simulink model "gg_plus_lc_platoon"  (R2019a)
settings: Solver=ode23t  StartTime=0.0  StopTime=70  FixedStep=0.1  MaxStep=0.01  RelTol=1e-3
InitFcn:
  | load vehStatesBus
libraries: simulink x120, powerlib_meascontrol x14, dspsigops x7, autolibshared x7
(part 6 of 7)

== system gg_plus_lc_platoon/Lo/Regular Vehicle Following/Compute Errors ==
  xf : Inport
  vf : Inport  Port=2
  xl : Inport  Port=3
  vl : Inport  Port=4
  extraSpaceFlag : Inport  Port=5
  velFilterReset : Inport  Port=6
  Compare To Constant : simulink/Logic and Bit Operations/Compare To Constant  relop=<  const=-0.1  OutDataTypeStr=boolean
  Demux : Demux  Outputs=2
  Demux1 : Demux  Outputs=2
  Gain3 : Gain  Gain=velFilterGain
  Integrator : Integrator  InitialCondition=[h d0]
  Integrator1 : Integrator  ExternalReset=rising  InitialCondition=vx0
  Multiply : Product
  Mux : Mux  Inputs=2
  Mux1 : Mux  Inputs=2
  Product : Product
  Saturation : Saturate  UpperLimit=maxAcceleration  LowerLimit=minAcceleration
  Saturation1 : Saturate  UpperLimit=hFilterSaturation  LowerLimit=-hFilterSaturation
  Sum : Sum  Inputs=-+|
  Sum1 : Sum  Inputs=++|
  Sum2 : Sum  Inputs=+-|
  Sum3 : Sum  Inputs=|++
  Sum4 : Sum  Inputs=-+|
  Sum5 : Sum  Inputs=|+-
  Sum6 : Sum  Inputs=+-|
  Sum7 : Sum  Inputs=|++
  Sum8 : Sum  Inputs=|+-
  Switch : Switch  Criteria=u2 > Threshold
  d0 : Constant  Value=d0
  d0Lc : Constant  Value=d0Lc
  h : Constant  Value=h
  hFilterGain : Gain  Gain=hFilterGain
  hLc : Constant  Value=hLc
  vLen : Constant  Value=lr+lf
  eh : Outport
  ev : Outport  Port=2
  "gap " : Outport  Port=3
  unsafeFlag : Outport  Port=4
  wires:
  Sum8/1 -> Gain3/1
  Integrator1/1 -> Sum4/2, Sum8/2
  Saturation/1 -> Integrator1/1
  Gain3/1 -> Saturation/1
  Sum4/1 -> ev/1
  vl/1 -> Sum8/1
  d0Lc/1 -> Mux1/2
  hFilterGain/1 -> Saturation1/1
  Demux/1 -> Multiply/2
  xf/1 -> Sum1/2
  Sum/1 -> Sum2/1, "gap "/1, Sum6/1  "gap"
  Multiply/1 -> Sum3/1
  Demux1/2 -> Sum7/2
  hLc/1 -> Mux1/1
  vLen/1 -> Sum1/1
  Demux/2 -> Sum3/2
  Switch/1 -> Sum5/1
  Sum5/1 -> hFilterGain/1
  vf/1 -> Multiply/1, Product/1, Sum4/1
  Sum1/1 -> Sum/1  "x (front bumber)"
  Sum3/1 -> Sum2/2  "desired  gap"
  h/1 -> Mux/1
  Product/1 -> Sum7/1
  xl/1 -> Sum/2
  extraSpaceFlag/1 -> Switch/2
  Sum2/1 -> eh/1
  Compare To Constant/1 -> unsafeFlag/1
  Demux1/1 -> Product/2
  Integrator/1 -> Sum5/2, Demux/1
  d0/1 -> Mux/2
  Mux1/1 -> Switch/1
  Sum7/1 -> Sum6/2  "safe  gap"
  Mux/1 -> Demux1/1, Switch/3  "min safe gap"
  Sum6/1 -> Compare To Constant/1
  velFilterReset/1 -> Integrator1/2
  Saturation1/1 -> Integrator/1

== system gg_plus_lc_platoon/Lo/Regular Vehicle Following/Veh Following ==
  eh : Inport
  ev : Inport  Port=2
  realInput : Inport  Port=3
  intReset : Inport  Port=4
  Anti-windup gain : Gain  Gain=sqrt(Ki/Kd)
  Integrator : Integrator  ExternalReset=rising
  Kd : Gain  Gain=Kd
  Ki : Gain  Gain=Ki
  Kp : Gain  Gain=Kp
  Saturation1 : Saturate  UpperLimit=maxHeadwayError  LowerLimit=minHeadwayError
  Scope : Scope  NumInputPorts=4
  Sum : Sum  Inputs=|-+
  Sum1 : Sum  Inputs=+++
  Sum5 : Sum  Inputs=-+|
  u : Outport
  wires:
  intReset/1 -> Integrator/2
  ev/1 -> Kd/1
  Ki/1 -> Sum5/2
  Anti-windup gain/1 -> Sum5/1
  Sum5/1 -> Integrator/1
  Kp/1 -> Sum1/2, Scope/2
  Kd/1 -> Sum1/3, Scope/3
  Saturation1/1 -> Ki/1, Kp/1
  eh/1 -> Saturation1/1
  Sum1/1 -> u/1, Sum/2, Scope/4
  realInput/1 -> Sum/1
  Sum/1 -> Anti-windup gain/1
  Integrator/1 -> Scope/1, Sum1/1

== system gg_plus_lc_platoon/Lo/Regular Vehicle Following/Velocity Control ==
  velocity : Inport
  realInput : Inport  Port=2
  intReset : Inport  Port=3
  Anti-windup gain : Gain  Gain=velKp/velKi
  Integrator2 : Integrator  ExternalReset=falling
  Sum : Sum  Inputs=|+-
  Sum1 : Sum  Inputs=|-+
  Sum2 : Sum  Inputs=-+|
  Sum3 : Sum  Inputs=|++
  freeFlowVel : Constant  Value=freeFlowVel
  velKi : Gain  Gain=velKi
  velKp : Gain  Gain=velKp
  u : Outport
  wires:
  Anti-windup gain/1 -> Sum2/1
  Sum/1 -> velKi/1, velKp/1
  velKp/1 -> Sum3/2
  velKi/1 -> Sum2/2
  Integrator2/1 -> Sum3/1
  velocity/1 -> Sum/2
  freeFlowVel/1 -> Sum/1
  intReset/1 -> Integrator2/2
  Sum3/1 -> Sum1/2, u/1
  realInput/1 -> Sum1/1
  Sum1/1 -> Anti-windup gain/1
  Sum2/1 -> Integrator2/1

== system gg_plus_lc_platoon/Lo/Subsystem1/Triggered Subsystem1 ==
  Trigger : TriggerPort  VariantControl=Variant
  Constant : Constant  Value=true  OutDataTypeStr=boolean
  Out1 : Outport  OutDataTypeStr=boolean  InitialOutput=0
  wires:
  Constant/1 -> Out1/1

== system gg_plus_lc_platoon/Lo/Subsystem1/safeErrors1 ==
  errors : Inport
  AND : Logic  IconShape=distinctive  AllPortsSameDT=off  OutDataTypeStr=boolean
  Compare To Constant4 : simulink/Logic and Bit Operations/Compare To Constant  relop=>=  const=-0.1  OutDataTypeStr=boolean
  Demux : Demux  Outputs=2
  safetyFlag : Outport
  wires:
  Compare To Constant4/1 -> Demux/1
  errors/1 -> Compare To Constant4/1
  AND/1 -> safetyFlag/1
  Demux/1 -> AND/1
  Demux/2 -> AND/2

== system gg_plus_lc_platoon/Lo/Subsystem1/safeErrors2 ==
  errors : Inport
  AND : Logic  IconShape=distinctive  AllPortsSameDT=off  OutDataTypeStr=boolean
  Compare To Constant4 : simulink/Logic and Bit Operations/Compare To Constant  relop=>=  const=-0.1  OutDataTypeStr=boolean
  Demux : Demux  Outputs=2
  safetyFlag : Outport
  wires:
  Demux/2 -> AND/2
  Demux/1 -> AND/1
  AND/1 -> safetyFlag/1
  errors/1 -> Compare To Constant4/1
  Compare To Constant4/1 -> Demux/1

== system gg_plus_lc_platoon/Lo/Subsystem1/steadyState ==
  u : Inport
  AND : Logic  IconShape=distinctive  AllPortsSameDT=off  OutDataTypeStr=boolean
  Abs2 : Abs
  Compare To Constant2 : simulink/Logic and Bit Operations/Compare To Constant  relop=<=  const=0.2  OutDataTypeStr=boolean
  Demux : Demux  Outputs=2
  Mux : Mux  Inputs=2
  Transport Delay2 : TransportDelay
  ssFlag : Outport
  wires:
  u/1 -> Transport Delay2/1, Mux/2
  Abs2/1 -> Compare To Constant2/1
  Demux/1 -> AND/1
  Transport Delay2/1 -> Mux/1
  AND/1 -> ssFlag/1
  Compare To Constant2/1 -> Demux/1
  Mux/1 -> Abs2/1
  Demux/2 -> AND/2

== system gg_plus_lc_platoon/Lo/Virtual Vehicle Following/Compute Errors ==
  xf : Inport
  vf : Inport  Port=2
  xl : Inport  Port=3
  vl : Inport  Port=4
  extraSpace : Inport  Port=5
  velFilterReset : Inport  Port=6
  Compare To Constant : simulink/Logic and Bit Operations/Compare To Constant  relop=<=  const=0  OutDataTypeStr=boolean
  Demux : Demux  Outputs=2
  Demux1 : Demux  Outputs=2
  Gain3 : Gain  Gain=velFilterGain/10
  Integrator : Integrator  InitialCondition=[h d0]
  Integrator1 : Integrator  ExternalReset=rising  InitialCondition=vx0
  Multiply : Product
  Mux : Mux  Inputs=2
  Mux1 : Mux  Inputs=2
  Product : Product
  Saturation : Saturate  UpperLimit=maxAcceleration  LowerLimit=minAcceleration
  Saturation1 : Saturate  UpperLimit=hFilterSaturation  LowerLimit=-hFilterSaturation
  Sum : Sum  Inputs=-+|
  Sum1 : Sum  Inputs=++|
  Sum2 : Sum  Inputs=+-|
  Sum3 : Sum  Inputs=|++
  Sum4 : Sum  Inputs=-+|
  Sum5 : Sum  Inputs=|+-
  Sum6 : Sum  Inputs=+-|
  Sum7 : Sum  Inputs=|++
  Sum8 : Sum  Inputs=|+-
  Switch : Switch  Criteria=u2 > Threshold
  d0 : Constant  Value=d0
  d0Lc : Constant  Value=d0Lc
  h : Constant  Value=h
  hFilterGain : Gain  Gain=hFilterGain
  hLc : Constant  Value=hLc
  vLen : Constant  Value=lr+lf
  eh : Outport
  ev : Outport  Port=2
  "gap " : Outport  Port=3
  unsafeFlag : Outport  Port=4
  wires:
  velFilterReset/1 -> Integrator1/2
  xl/1 -> Sum/2
  Sum6/1 -> Compare To Constant/1
  Mux/1 -> Demux1/1, Switch/3  "min safe gap"
  Sum7/1 -> Sum6/2  "safe  gap"
  Mux1/1 -> Switch/1
  d0/1 -> Mux/2
  Integrator/1 -> Demux/1, Sum5/2
  Demux1/1 -> Product/2
  Compare To Constant/1 -> unsafeFlag/1
  Sum2/1 -> eh/1
  extraSpace/1 -> Switch/2
  Product/1 -> Sum7/1
  h/1 -> Mux/1
  Sum3/1 -> Sum2/2  "desired  gap"
  Sum1/1 -> Sum/1  "x (front bumber)"
  vf/1 -> Sum4/1, Product/1, Multiply/1
  Sum5/1 -> hFilterGain/1
  Switch/1 -> Sum5/1
  Demux/2 -> Sum3/2
  vLen/1 -> Sum1/1
  hLc/1 -> Mux1/1
  Demux1/2 -> Sum7/2
  Multiply/1 -> Sum3/1
  Sum/1 -> Sum6/1, "gap "/1, Sum2/1  "gap"
  xf/1 -> Sum1/2
  Demux/1 -> Multiply/2
  hFilterGain/1 -> Saturation1/1
  d0Lc/1 -> Mux1/2
  Sum4/1 -> ev/1
  Integrator1/1 -> Sum4/2, Sum8/2
  Gain3/1 -> Saturation/1
  Sum8/1 -> Gain3/1
  Saturation/1 -> Integrator1/1
  vl/1 -> Sum8/1
  Saturation1/1 -> Integrator/1

== system gg_plus_lc_platoon/Lo/Virtual Vehicle Following/Velocity Control Free Flow ==
  ev : Inport
  realInput : Inport  Port=2
  intReset : Inport  Port=3
  Anti-windup gain : Gain  Gain=velKp/velKi
  Integrator2 : Integrator  ExternalReset=falling
  Sum1 : Sum  Inputs=|-+
  Sum2 : Sum  Inputs=-+|
  Sum3 : Sum  Inputs=|++
  velKi : Gain  Gain=velKi
  velKp : Gain  Gain=velKp
  u : Outport
  wires:
  Sum2/1 -> Integrator2/1
  Sum1/1 -> Anti-windup gain/1
  realInput/1 -> Sum1/1
  Anti-windup gain/1 -> Sum2/1
  Sum3/1 -> u/1, Sum1/2
  intReset/1 -> Integrator2/2
  Integrator2/1 -> Sum3/1
  velKi/1 -> Sum2/2
  velKp/1 -> Sum3/2
  ev/1 -> velKp/1, velKi/1

== system gg_plus_lc_platoon/Lo/Virtual Vehicle Following/Velocity Control Min ==
  note: Velocity control
  ev : Inport
  intReset : Inport  Port=2
  Integrator2 : Integrator  ExternalReset=rising
  Sum3 : Sum
  velKi : Gain  Gain=velKi
  velKp : Gain  Gain=velKp
  u : Outport
  wires:
  Integrator2/1 -> velKi/1
  velKi/1 -> Sum3/2
  Sum3/1 -> u/1
  velKp/1 -> Sum3/1
  ev/1 -> velKp/1, Integrator2/1
  intReset/1 -> Integrator2/2

== system gg_plus_lc_platoon/Lo/Virtual Vehicle Following/Virtual Leader Following ==
  eh : Inport
  ev : Inport  Port=2
  realInput : Inport  Port=3
  intReset : Inport  Port=4
  Anti-windup gain : Gain  Gain=sqrt(Ki/Kd)
  Gain : Gain  Gain=10
  Integrator : Integrator  ExternalReset=rising
  Integrator2 : Integrator  ExternalReset=rising
  Kd : Gain  Gain=Kd
  Ki : Gain  Gain=Ki
  Kp : Gain  Gain=Kp
  Saturation1 : Saturate  UpperLimit=maxHeadwayError  LowerLimit=minHeadwayError
  Scope : Scope  NumInputPorts=4
  Scope1 : Scope  NumInputPorts=2
  Sum : Sum  Inputs=|-+
  Sum1 : Sum  Inputs=+++
  Sum5 : Sum  Inputs=-+|
  Sum9 : Sum  Inputs=|+-
  u : Outport
  wires:
  Saturation1/1 -> Sum9/1, Scope1/1
  Sum9/1 -> Gain/1
  Gain/1 -> Integrator2/1
  ev/1 -> Kd/1
  Ki/1 -> Sum5/2
  Anti-windup gain/1 -> Sum5/1
  Sum5/1 -> Integrator/1
  Integrator/1 -> Sum1/1, Scope/1
  Kp/1 -> Scope/2, Sum1/2
  Kd/1 -> Scope/3, Sum1/3
  Integrator2/1 -> Kp/1, Ki/1, Scope1/2, Sum9/2
  eh/1 -> Saturation1/1
  Sum1/1 -> Sum/2, u/1, Scope/4
  realInput/1 -> Sum/1
  Sum/1 -> Anti-windup gain/1
  intReset/1 -> Integrator/2, Integrator2/2

== system gg_plus_lc_platoon/Lo/findLeader/Subsystem ==
  ego : Inport
  all : Inport  Port=2
  Enable : EnablePort
  MATLAB Function : MATLAB Function  TreatAsAtomicUnit=on
  idx : Outport  InitialOutput=1
  wires:
  ego/1 -> MATLAB Function/1(ego)
  MATLAB Function/1(leaderIdx) -> idx/1
  all/1 -> MATLAB Function/2(allVehicles)

== system gg_plus_lc_platoon/Lo/findLeader/farAwayVeh ==
  ego : Inport  OutDataTypeStr=Bus: vehStatesBus
  Bus Creator : BusCreator  Inputs=6  OutDataTypeStr=Bus: vehStatesBus  NonVirtualBus=on
  Bus Selector : BusSelector  OutputSignals=X,Y,Xdot,psi,u,delta
  Constant : Constant  Value=1000
  Sum : Sum  Inputs=++|
  Out1 : Outport  OutDataTypeStr=Bus: vehStatesBus
  wires:
  Bus Creator/1 -> Out1/1
  Constant/1 -> Sum/1
  Bus Selector/1 -> Sum/2  "<X>"
  ego/1 -> Bus Selector/1
  Sum/1 -> Bus Creator/1  "X"
  Bus Selector/2 -> Bus Creator/2  "<Y>"
  Bus Selector/3 -> Bus Creator/3  "<Xdot>"
  Bus Selector/4 -> Bus Creator/4  "<psi>"
  Bus Selector/5 -> Bus Creator/5  "<u>"
  Bus Selector/6 -> Bus Creator/6  "<delta>"

== system gg_plus_lc_platoon/Lo/followerErrors/gapToFollower ==
  xf : Inport
  vf : Inport  Port=2
  xl : Inport  Port=3
  Multiply : Product
  Sum : Sum  Inputs=-+|
  Sum1 : Sum  Inputs=++|
  Sum2 : Sum  Inputs=+-|
  Sum3 : Sum  Inputs=|++
  d0 : Constant  Value=d0
  h : Constant  Value=h
  vLen : Constant  Value=lr+lf
  eh : Outport
  "gap " : Outport  Port=2
  wires:
  vLen/1 -> Sum1/1
  Multiply/1 -> Sum3/1
  Sum/1 -> "gap "/1, Sum2/1  "gap"
  xf/1 -> Sum1/2
  Sum3/1 -> Sum2/2  "desired  gap"
  vf/1 -> Multiply/1
  Sum1/1 -> Sum/1  "x (front bumber)"
  xl/1 -> Sum/2
  Sum2/1 -> eh/1
  h/1 -> Multiply/2  "time headway"
  d0/1 -> Sum3/2  "gap at  standstill"

== system gg_plus_lc_platoon/Lo/safeErrors/Triggered Subsystem1 ==
  Trigger : TriggerPort  VariantControl=Variant
  Constant : Constant  Value=true  OutDataTypeStr=boolean
  Out1 : Outport  OutDataTypeStr=boolean  InitialOutput=0
  wires:
  Constant/1 -> Out1/1

== system gg_plus_lc_platoon/p1/Lateral Control/Full State Observer ==
  note: xhat
  note: yhat
  measuredOutputs : Inport
  delta : Inport  Port=2
  Add1 : Sum  Inputs=|-+
  Gain : Gain  Gain=B  Multiplication=Matrix(K*u)
  Gain1 : Gain  Gain=C  Multiplication=Matrix(K*u)
  Gain2 : Gain  Gain=L  Multiplication=Matrix(K*u)
  Gain3 : Gain  Gain=A  Multiplication=Matrix(K*u)
  Integrator : Integrator  InitialCondition=[y0; 0; 0; 0]
  Signal Specification : SignalSpecification  Dimensions=[size(C,1) 1]
  Sum : Sum  Inputs=+++
  xhat : Outport
  wires:
  Add1/1 -> Signal Specification/1
  Integrator/1 -> xhat/1, Gain3/1, Gain1/1
  Gain1/1 -> Add1/1
  Sum/1 -> Integrator/1
  measuredOutputs/1 -> Add1/2
  delta/1 -> Gain/1
  Gain/1 -> Sum/3
  Gain3/1 -> Sum/2
  Signal Specification/1 -> Gain2/1
  Gain2/1 -> Sum/1

== system gg_plus_lc_platoon/p1/Lateral Control/Triggered Subsystem1 ==
  In1 : Inport
  Trigger : TriggerPort  VariantControl=Variant
  Out1 : Outport  InitialOutput=y0
  wires:
  In1/1 -> Out1/1

== system gg_plus_lc_platoon/p1/Regular Vehicle Following/Compute Errors ==
  xf : Inport
  vf : Inport  Port=2
  xl : Inport  Port=3
  vl : Inport  Port=4
  extraSpaceFlag : Inport  Port=5
  velFilterReset : Inport  Port=6
  Compare To Constant : simulink/Logic and Bit Operations/Compare To Constant  relop=<  const=-0.1  OutDataTypeStr=boolean
  Demux : Demux  Outputs=2
  Demux1 : Demux  Outputs=2
  Gain3 : Gain  Gain=velFilterGain
  Integrator : Integrator  InitialCondition=[h d0]
  Integrator1 : Integrator  ExternalReset=rising  InitialCondition=vx0
  Multiply : Product
  Mux : Mux  Inputs=2
  Mux1 : Mux  Inputs=2
  Product : Product
  Saturation : Saturate  UpperLimit=maxAcceleration  LowerLimit=minAcceleration
  Saturation1 : Saturate  UpperLimit=hFilterSaturation  LowerLimit=-hFilterSaturation
  Sum : Sum  Inputs=-+|
  Sum1 : Sum  Inputs=++|
  Sum2 : Sum  Inputs=+-|
  Sum3 : Sum  Inputs=|++
  Sum4 : Sum  Inputs=-+|
  Sum5 : Sum  Inputs=|+-
  Sum6 : Sum  Inputs=+-|
  Sum7 : Sum  Inputs=|++
  Sum8 : Sum  Inputs=|+-
  Switch : Switch  Criteria=u2 > Threshold
  d0 : Constant  Value=d0
  d0Lc : Constant  Value=d0Lc
  h : Constant  Value=h
  hFilterGain : Gain  Gain=hFilterGain
  hLc : Constant  Value=hLc
  vLen : Constant  Value=lr+lf
  eh : Outport
  ev : Outport  Port=2
  "gap " : Outport  Port=3
  unsafeFlag : Outport  Port=4
  wires:
  Saturation1/1 -> Integrator/1
  velFilterReset/1 -> Integrator1/2
  Sum6/1 -> Compare To Constant/1
  Mux/1 -> Switch/3, Demux1/1  "min safe gap"
  Sum7/1 -> Sum6/2  "safe  gap"
  Mux1/1 -> Switch/1
  d0/1 -> Mux/2
  Integrator/1 -> Demux/1, Sum5/2
  Demux1/1 -> Product/2
  Compare To Constant/1 -> unsafeFlag/1
  Sum2/1 -> eh/1
  extraSpaceFlag/1 -> Switch/2
  xl/1 -> Sum/2
  Product/1 -> Sum7/1
  h/1 -> Mux/1
  Sum3/1 -> Sum2/2  "desired  gap"
  Sum1/1 -> Sum/1  "x (front bumber)"
  vf/1 -> Sum4/1, Product/1, Multiply/1
  Sum5/1 -> hFilterGain/1
  Switch/1 -> Sum5/1
  Demux/2 -> Sum3/2
  vLen/1 -> Sum1/1
  hLc/1 -> Mux1/1
  Demux1/2 -> Sum7/2
  Multiply/1 -> Sum3/1
  Sum/1 -> Sum6/1, "gap "/1, Sum2/1  "gap"
  xf/1 -> Sum1/2
  Demux/1 -> Multiply/2
  hFilterGain/1 -> Saturation1/1
  d0Lc/1 -> Mux1/2
  vl/1 -> Sum8/1
  Sum4/1 -> ev/1
  Gain3/1 -> Saturation/1
  Saturation/1 -> Integrator1/1
  Integrator1/1 -> Sum8/2, Sum4/2
  Sum8/1 -> Gain3/1

== system gg_plus_lc_platoon/p1/Regular Vehicle Following/Veh Following ==
  eh : Inport
  ev : Inport  Port=2
  realInput : Inport  Port=3
  intReset : Inport  Port=4
  Anti-windup gain : Gain  Gain=sqrt(Ki/Kd)
  Integrator : Integrator  ExternalReset=rising
  Kd : Gain  Gain=Kd
  Ki : Gain  Gain=Ki
  Kp : Gain  Gain=Kp
  Saturation1 : Saturate  UpperLimit=maxHeadwayError  LowerLimit=minHeadwayError
  Scope : Scope  NumInputPorts=4
  Sum : Sum  Inputs=|-+
  Sum1 : Sum  Inputs=+++
  Sum5 : Sum  Inputs=-+|
  u : Outport
  wires:
  Integrator/1 -> Sum1/1, Scope/1
  Sum/1 -> Anti-windup gain/1
  realInput/1 -> Sum/1
  Sum1/1 -> Scope/4, Sum/2, u/1
  eh/1 -> Saturation1/1
  Saturation1/1 -> Kp/1, Ki/1
  Kd/1 -> Scope/3, Sum1/3
  Kp/1 -> Scope/2, Sum1/2
  Sum5/1 -> Integrator/1
  Anti-windup gain/1 -> Sum5/1
  Ki/1 -> Sum5/2
  ev/1 -> Kd/1
  intReset/1 -> Integrator/2

== system gg_plus_lc_platoon/p1/Regular Vehicle Following/Velocity Control ==
  velocity : Inport
  realInput : Inport  Port=2
  intReset : Inport  Port=3
  Anti-windup gain : Gain  Gain=velKp/velKi
  Integrator2 : Integrator  ExternalReset=falling
  Sum : Sum  Inputs=|+-
  Sum1 : Sum  Inputs=|-+
  Sum2 : Sum  Inputs=-+|
  Sum3 : Sum  Inputs=|++
  freeFlowVel : Constant  Value=freeFlowVel
  velKi : Gain  Gain=velKi
  velKp : Gain  Gain=velKp
  u : Outport
  wires:
  Sum2/1 -> Integrator2/1
  Sum1/1 -> Anti-windup gain/1
  realInput/1 -> Sum1/1
  Sum3/1 -> u/1, Sum1/2
  intReset/1 -> Integrator2/2
  freeFlowVel/1 -> Sum/1
  velocity/1 -> Sum/2
  Integrator2/1 -> Sum3/1
  velKi/1 -> Sum2/2
  velKp/1 -> Sum3/2
  Sum/1 -> velKp/1, velKi/1
  Anti-windup gain/1 -> Sum2/1

== system gg_plus_lc_platoon/p1/Subsystem1/Triggered Subsystem1 ==
  Trigger : TriggerPort  VariantControl=Variant
  Constant : Constant  Value=true  OutDataTypeStr=boolean
  Out1 : Outport  OutDataTypeStr=boolean  InitialOutput=0
  wires:
  Constant/1 -> Out1/1

== system gg_plus_lc_platoon/p1/Subsystem1/safeErrors1 ==
  errors : Inport
  AND : Logic  IconShape=distinctive  AllPortsSameDT=off  OutDataTypeStr=boolean
  Compare To Constant4 : simulink/Logic and Bit Operations/Compare To Constant  relop=>=  const=-0.1  OutDataTypeStr=boolean
  Demux : Demux  Outputs=2
  safetyFlag : Outport
  wires:
  Demux/2 -> AND/2
  Demux/1 -> AND/1
  AND/1 -> safetyFlag/1
  errors/1 -> Compare To Constant4/1
  Compare To Constant4/1 -> Demux/1

== system gg_plus_lc_platoon/p1/Subsystem1/safeErrors2 ==
  errors : Inport
  AND : Logic  IconShape=distinctive  AllPortsSameDT=off  OutDataTypeStr=boolean
  Compare To Constant4 : simulink/Logic and Bit Operations/Compare To Constant  relop=>=  const=-0.1  OutDataTypeStr=boolean
  Demux : Demux  Outputs=2
  safetyFlag : Outport
  wires:
  Compare To Constant4/1 -> Demux/1
  errors/1 -> Compare To Constant4/1
  AND/1 -> safetyFlag/1
  Demux/1 -> AND/1
  Demux/2 -> AND/2

== system gg_plus_lc_platoon/p1/Subsystem1/steadyState ==
  u : Inport
  AND : Logic  IconShape=distinctive  AllPortsSameDT=off  OutDataTypeStr=boolean
  Abs2 : Abs
  Compare To Constant2 : simulink/Logic and Bit Operations/Compare To Constant  relop=<=  const=0.2  OutDataTypeStr=boolean
  Demux : Demux  Outputs=2
  Mux : Mux  Inputs=2
  Transport Delay2 : TransportDelay
  ssFlag : Outport
  wires:
  Demux/2 -> AND/2
  Mux/1 -> Abs2/1
  Compare To Constant2/1 -> Demux/1
  AND/1 -> ssFlag/1
  Transport Delay2/1 -> Mux/1
  Demux/1 -> AND/1
  Abs2/1 -> Compare To Constant2/1
  u/1 -> Mux/2, Transport Delay2/1

== system gg_plus_lc_platoon/p1/Virtual Vehicle Following/Compute Errors ==
  xf : Inport
  vf : Inport  Port=2
  xl : Inport  Port=3
  vl : Inport  Port=4
  extraSpace : Inport  Port=5
  velFilterReset : Inport  Port=6
  Compare To Constant : simulink/Logic and Bit Operations/Compare To Constant  relop=<=  const=0  OutDataTypeStr=boolean
  Demux : Demux  Outputs=2
  Demux1 : Demux  Outputs=2
  Gain3 : Gain  Gain=velFilterGain/10
  Integrator : Integrator  InitialCondition=[h d0]
  Integrator1 : Integrator  ExternalReset=rising  InitialCondition=vx0
  Multiply : Product
  Mux : Mux  Inputs=2
  Mux1 : Mux  Inputs=2
  Product : Product
  Saturation : Saturate  UpperLimit=maxAcceleration  LowerLimit=minAcceleration
  Saturation1 : Saturate  UpperLimit=hFilterSaturation  LowerLimit=-hFilterSaturation
  Sum : Sum  Inputs=-+|
  Sum1 : Sum  Inputs=++|
  Sum2 : Sum  Inputs=+-|
  Sum3 : Sum  Inputs=|++
  Sum4 : Sum  Inputs=-+|
  Sum5 : Sum  Inputs=|+-
  Sum6 : Sum  Inputs=+-|
  Sum7 : Sum  Inputs=|++
  Sum8 : Sum  Inputs=|+-
  Switch : Switch  Criteria=u2 > Threshold
  d0 : Constant  Value=d0
  d0Lc : Constant  Value=d0Lc
  h : Constant  Value=h
  hFilterGain : Gain  Gain=hFilterGain
  hLc : Constant  Value=hLc
  vLen : Constant  Value=lr+lf
  eh : Outport
  ev : Outport  Port=2
  "gap " : Outport  Port=3
  unsafeFlag : Outport  Port=4
  wires:
  Saturation1/1 -> Integrator/1
  vl/1 -> Sum8/1
  Saturation/1 -> Integrator1/1
  Sum8/1 -> Gain3/1
  Gain3/1 -> Saturation/1
  Integrator1/1 -> Sum8/2, Sum4/2
  Sum4/1 -> ev/1
  d0Lc/1 -> Mux1/2
  hFilterGain/1 -> Saturation1/1
  Demux/1 -> Multiply/2
  xf/1 -> Sum1/2
  Sum/1 -> Sum2/1, "gap "/1, Sum6/1  "gap"
  Multiply/1 -> Sum3/1
  Demux1/2 -> Sum7/2
  hLc/1 -> Mux1/1
  vLen/1 -> Sum1/1
  Demux/2 -> Sum3/2
  Switch/1 -> Sum5/1
  Sum5/1 -> hFilterGain/1
  vf/1 -> Multiply/1, Product/1, Sum4/1
  Sum1/1 -> Sum/1  "x (front bumber)"
  Sum3/1 -> Sum2/2  "desired  gap"
  h/1 -> Mux/1
  Product/1 -> Sum7/1
  extraSpace/1 -> Switch/2
  Sum2/1 -> eh/1
  Compare To Constant/1 -> unsafeFlag/1
  Demux1/1 -> Product/2
  Integrator/1 -> Sum5/2, Demux/1
  d0/1 -> Mux/2
  Mux1/1 -> Switch/1
  Sum7/1 -> Sum6/2  "safe  gap"
  Mux/1 -> Switch/3, Demux1/1  "min safe gap"
  Sum6/1 -> Compare To Constant/1
  xl/1 -> Sum/2
  velFilterReset/1 -> Integrator1/2

== system gg_plus_lc_platoon/p1/Virtual Vehicle Following/Velocity Control Free Flow ==
  ev : Inport
  realInput : Inport  Port=2
  intReset : Inport  Port=3
  Anti-windup gain : Gain  Gain=velKp/velKi
  Integrator2 : Integrator  ExternalReset=falling
  Sum1 : Sum  Inputs=|-+
  Sum2 : Sum  Inputs=-+|
  Sum3 : Sum  Inputs=|++
  velKi : Gain  Gain=velKi
  velKp : Gain  Gain=velKp
  u : Outport
  wires:
  ev/1 -> velKi/1, velKp/1
  velKp/1 -> Sum3/2
  velKi/1 -> Sum2/2
  Integrator2/1 -> Sum3/1
  intReset/1 -> Integrator2/2
  Sum3/1 -> Sum1/2, u/1
  Anti-windup gain/1 -> Sum2/1
  realInput/1 -> Sum1/1
  Sum1/1 -> Anti-windup gain/1
  Sum2/1 -> Integrator2/1

== system gg_plus_lc_platoon/p1/Virtual Vehicle Following/Velocity Control Min ==
  note: Velocity control
  ev : Inport
  intReset : Inport  Port=2
  Integrator2 : Integrator  ExternalReset=rising
  Sum3 : Sum
  velKi : Gain  Gain=velKi
  velKp : Gain  Gain=velKp
  u : Outport
  wires:
  intReset/1 -> Integrator2/2
  ev/1 -> Integrator2/1, velKp/1
  velKp/1 -> Sum3/1
  Sum3/1 -> u/1
  velKi/1 -> Sum3/2
  Integrator2/1 -> velKi/1

== system gg_plus_lc_platoon/p1/Virtual Vehicle Following/Virtual Leader Following ==
  eh : Inport
  ev : Inport  Port=2
  realInput : Inport  Port=3
  intReset : Inport  Port=4
  Anti-windup gain : Gain  Gain=sqrt(Ki/Kd)
  Gain : Gain  Gain=10
  Integrator : Integrator  ExternalReset=rising
  Integrator2 : Integrator  ExternalReset=rising
  Kd : Gain  Gain=Kd
  Ki : Gain  Gain=Ki
  Kp : Gain  Gain=Kp
  Saturation1 : Saturate  UpperLimit=maxHeadwayError  LowerLimit=minHeadwayError
  Scope : Scope  NumInputPorts=4
  Scope1 : Scope  NumInputPorts=2
  Sum : Sum  Inputs=|-+
  Sum1 : Sum  Inputs=+++
  Sum5 : Sum  Inputs=-+|
  Sum9 : Sum  Inputs=|+-
  u : Outport
  wires:
  intReset/1 -> Integrator2/2, Integrator/2
  Sum/1 -> Anti-windup gain/1
  realInput/1 -> Sum/1
  Sum1/1 -> Scope/4, u/1, Sum/2
  eh/1 -> Saturation1/1
  Integrator2/1 -> Sum9/2, Scope1/2, Ki/1, Kp/1
  Kd/1 -> Sum1/3, Scope/3
  Kp/1 -> Sum1/2, Scope/2
  Integrator/1 -> Scope/1, Sum1/1
  Sum5/1 -> Integrator/1
  Anti-windup gain/1 -> Sum5/1
  Ki/1 -> Sum5/2
  ev/1 -> Kd/1
  Gain/1 -> Integrator2/1
  Sum9/1 -> Gain/1
  Saturation1/1 -> Scope1/1, Sum9/1

== system gg_plus_lc_platoon/p1/findLeader/Subsystem ==
  ego : Inport
  all : Inport  Port=2
  Enable : EnablePort
  MATLAB Function : MATLAB Function  TreatAsAtomicUnit=on
  idx : Outport  InitialOutput=1
  wires:
  all/1 -> MATLAB Function/2(allVehicles)
  MATLAB Function/1(leaderIdx) -> idx/1
  ego/1 -> MATLAB Function/1(ego)

== system gg_plus_lc_platoon/p1/findLeader/farAwayVeh ==
  ego : Inport  OutDataTypeStr=Bus: vehStatesBus
  Bus Creator : BusCreator  Inputs=6  OutDataTypeStr=Bus: vehStatesBus  NonVirtualBus=on
  Bus Selector : BusSelector  OutputSignals=X,Y,Xdot,psi,u,delta
  Constant : Constant  Value=1000
  Sum : Sum  Inputs=++|
  Out1 : Outport  OutDataTypeStr=Bus: vehStatesBus
  wires:
  Bus Selector/6 -> Bus Creator/6  "<delta>"
  Bus Selector/5 -> Bus Creator/5  "<u>"
  Bus Selector/4 -> Bus Creator/4  "<psi>"
  Bus Selector/3 -> Bus Creator/3  "<Xdot>"
  Bus Selector/2 -> Bus Creator/2  "<Y>"
  Sum/1 -> Bus Creator/1  "X"
  ego/1 -> Bus Selector/1
  Bus Selector/1 -> Sum/2  "<X>"
  Constant/1 -> Sum/1
  Bus Creator/1 -> Out1/1

== system gg_plus_lc_platoon/p1/followerErrors/gapToFollower ==
  xf : Inport
  vf : Inport  Port=2
  xl : Inport  Port=3
  Multiply : Product
  Sum : Sum  Inputs=-+|
  Sum1 : Sum  Inputs=++|
  Sum2 : Sum  Inputs=+-|
  Sum3 : Sum  Inputs=|++
  d0 : Constant  Value=d0
  h : Constant  Value=h
  vLen : Constant  Value=lr+lf
  eh : Outport
  "gap " : Outport  Port=2
  wires:
  d0/1 -> Sum3/2  "gap at  standstill"
  h/1 -> Multiply/2  "time headway"
  Sum2/1 -> eh/1
  xl/1 -> Sum/2
  Sum1/1 -> Sum/1  "x (front bumber)"
  vf/1 -> Multiply/1
  Sum3/1 -> Sum2/2  "desired  gap"
  xf/1 -> Sum1/2
  Sum/1 -> Sum2/1, "gap "/1  "gap"
  Multiply/1 -> Sum3/1
  vLen/1 -> Sum1/1

== system gg_plus_lc_platoon/p1/safeErrors/Triggered Subsystem1 ==
  Trigger : TriggerPort  VariantControl=Variant
  Constant : Constant  Value=true  OutDataTypeStr=boolean
  Out1 : Outport  OutDataTypeStr=boolean  InitialOutput=0
  wires:
  Constant/1 -> Out1/1

== system gg_plus_lc_platoon/p2/Lateral Control/Full State Observer ==
  note: yhat
  note: xhat
  measuredOutputs : Inport
  delta : Inport  Port=2
  Add1 : Sum  Inputs=|-+
  Gain : Gain  Gain=B  Multiplication=Matrix(K*u)
  Gain1 : Gain  Gain=C  Multiplication=Matrix(K*u)
  Gain2 : Gain  Gain=L  Multiplication=Matrix(K*u)
  Gain3 : Gain  Gain=A  Multiplication=Matrix(K*u)
  Integrator : Integrator  InitialCondition=[y0; 0; 0; 0]
  Signal Specification : SignalSpecification  Dimensions=[size(C,1) 1]
  Sum : Sum  Inputs=+++
  xhat : Outport
  wires:
  Gain2/1 -> Sum/1
  Signal Specification/1 -> Gain2/1
  Gain3/1 -> Sum/2
  Gain/1 -> Sum/3
  delta/1 -> Gain/1
  measuredOutputs/1 -> Add1/2
  Sum/1 -> Integrator/1
  Gain1/1 -> Add1/1
  Integrator/1 -> Gain1/1, Gain3/1, xhat/1
  Add1/1 -> Signal Specification/1

== system gg_plus_lc_platoon/p2/Lateral Control/Triggered Subsystem1 ==
  In1 : Inport
  Trigger : TriggerPort  VariantControl=Variant
  Out1 : Outport  InitialOutput=y0
  wires:
  In1/1 -> Out1/1

== system gg_plus_lc_platoon/p2/Regular Vehicle Following/Compute Errors ==
  xf : Inport
  vf : Inport  Port=2
  xl : Inport  Port=3
  vl : Inport  Port=4
  extraSpaceFlag : Inport  Port=5
  velFilterReset : Inport  Port=6
  Compare To Constant : simulink/Logic and Bit Operations/Compare To Constant  relop=<  const=-0.1  OutDataTypeStr=boolean
  Demux : Demux  Outputs=2
  Demux1 : Demux  Outputs=2
  Gain3 : Gain  Gain=velFilterGain
  Integrator : Integrator  InitialCondition=[h d0]
  Integrator1 : Integrator  ExternalReset=rising  InitialCondition=vx0
  Multiply : Product
  Mux : Mux  Inputs=2
  Mux1 : Mux  Inputs=2
  Product : Product
  Saturation : Saturate  UpperLimit=maxAcceleration  LowerLimit=minAcceleration
  Saturation1 : Saturate  UpperLimit=hFilterSaturation  LowerLimit=-hFilterSaturation
  Sum : Sum  Inputs=-+|
  Sum1 : Sum  Inputs=++|
  Sum2 : Sum  Inputs=+-|
  Sum3 : Sum  Inputs=|++
  Sum4 : Sum  Inputs=-+|
  Sum5 : Sum  Inputs=|+-
  Sum6 : Sum  Inputs=+-|
  Sum7 : Sum  Inputs=|++
  Sum8 : Sum  Inputs=|+-
  Switch : Switch  Criteria=u2 > Threshold
  d0 : Constant  Value=d0
  d0Lc : Constant  Value=d0Lc
  h : Constant  Value=h
  hFilterGain : Gain  Gain=hFilterGain
  hLc : Constant  Value=hLc
  vLen : Constant  Value=lr+lf
  eh : Outport
  ev : Outport  Port=2
  "gap " : Outport  Port=3
  unsafeFlag : Outport  Port=4
  wires:
  Sum8/1 -> Gain3/1
  Integrator1/1 -> Sum4/2, Sum8/2
  Saturation/1 -> Integrator1/1
  Gain3/1 -> Saturation/1
  Sum4/1 -> ev/1
  vl/1 -> Sum8/1
  d0Lc/1 -> Mux1/2
  hFilterGain/1 -> Saturation1/1
  Demux/1 -> Multiply/2
  xf/1 -> Sum1/2
  Sum/1 -> Sum2/1, "gap "/1, Sum6/1  "gap"
  Multiply/1 -> Sum3/1
  Demux1/2 -> Sum7/2
  hLc/1 -> Mux1/1
  vLen/1 -> Sum1/1
  Demux/2 -> Sum3/2
  Switch/1 -> Sum5/1
  Sum5/1 -> hFilterGain/1
  vf/1 -> Multiply/1, Product/1, Sum4/1
  Sum1/1 -> Sum/1  "x (front bumber)"
  Sum3/1 -> Sum2/2  "desired  gap"
  h/1 -> Mux/1
  Product/1 -> Sum7/1
  xl/1 -> Sum/2
  extraSpaceFlag/1 -> Switch/2
  Sum2/1 -> eh/1
  Compare To Constant/1 -> unsafeFlag/1
  Demux1/1 -> Product/2
  Integrator/1 -> Sum5/2, Demux/1
  d0/1 -> Mux/2
  Mux1/1 -> Switch/1
  Sum7/1 -> Sum6/2  "safe  gap"
  Mux/1 -> Demux1/1, Switch/3  "min safe gap"
  Sum6/1 -> Compare To Constant/1
  velFilterReset/1 -> Integrator1/2
  Saturation1/1 -> Integrator/1

== system gg_plus_lc_platoon/p2/Regular Vehicle Following/Veh Following ==
  eh : Inport
  ev : Inport  Port=2
  realInput : Inport  Port=3
  intReset : Inport  Port=4
  Anti-windup gain : Gain  Gain=sqrt(Ki/Kd)
  Integrator : Integrator  ExternalReset=rising
  Kd : Gain  Gain=Kd
  Ki : Gain  Gain=Ki
  Kp : Gain  Gain=Kp
  Saturation1 : Saturate  UpperLimit=maxHeadwayError  LowerLimit=minHeadwayError
  Scope : Scope  NumInputPorts=4
  Sum : Sum  Inputs=|-+
  Sum1 : Sum  Inputs=+++
  Sum5 : Sum  Inputs=-+|
  u : Outport
  wires:
  intReset/1 -> Integrator/2
  ev/1 -> Kd/1
  Ki/1 -> Sum5/2
  Anti-windup gain/1 -> Sum5/1
  Sum5/1 -> Integrator/1
  Kp/1 -> Sum1/2, Scope/2
  Kd/1 -> Sum1/3, Scope/3
  Saturation1/1 -> Ki/1, Kp/1
  eh/1 -> Saturation1/1
  Sum1/1 -> u/1, Sum/2, Scope/4
  realInput/1 -> Sum/1
  Sum/1 -> Anti-windup gain/1
  Integrator/1 -> Scope/1, Sum1/1

== system gg_plus_lc_platoon/p2/Regular Vehicle Following/Velocity Control ==
  velocity : Inport
  realInput : Inport  Port=2
  intReset : Inport  Port=3
  Anti-windup gain : Gain  Gain=velKp/velKi
  Integrator2 : Integrator  ExternalReset=falling
  Sum : Sum  Inputs=|+-
  Sum1 : Sum  Inputs=|-+
  Sum2 : Sum  Inputs=-+|
  Sum3 : Sum  Inputs=|++
  freeFlowVel : Constant  Value=freeFlowVel
  velKi : Gain  Gain=velKi
  velKp : Gain  Gain=velKp
  u : Outport
  wires:
  Anti-windup gain/1 -> Sum2/1
  Sum/1 -> velKi/1, velKp/1
  velKp/1 -> Sum3/2
  velKi/1 -> Sum2/2
  Integrator2/1 -> Sum3/1
  velocity/1 -> Sum/2
  freeFlowVel/1 -> Sum/1
  intReset/1 -> Integrator2/2
  Sum3/1 -> Sum1/2, u/1
  realInput/1 -> Sum1/1
  Sum1/1 -> Anti-windup gain/1
  Sum2/1 -> Integrator2/1

== system gg_plus_lc_platoon/p2/Subsystem1/Triggered Subsystem1 ==
  Trigger : TriggerPort  VariantControl=Variant
  Constant : Constant  Value=true  OutDataTypeStr=boolean
  Out1 : Outport  OutDataTypeStr=boolean  InitialOutput=0
  wires:
  Constant/1 -> Out1/1

== system gg_plus_lc_platoon/p2/Subsystem1/safeErrors1 ==
  errors : Inport
  AND : Logic  IconShape=distinctive  AllPortsSameDT=off  OutDataTypeStr=boolean
  Compare To Constant4 : simulink/Logic and Bit Operations/Compare To Constant  relop=>=  const=-0.1  OutDataTypeStr=boolean
  Demux : Demux  Outputs=2
  safetyFlag : Outport
  wires:
  Compare To Constant4/1 -> Demux/1
  errors/1 -> Compare To Constant4/1
  AND/1 -> safetyFlag/1
  Demux/1 -> AND/1
  Demux/2 -> AND/2

== system gg_plus_lc_platoon/p2/Subsystem1/safeErrors2 ==
  errors : Inport
  AND : Logic  IconShape=distinctive  AllPortsSameDT=off  OutDataTypeStr=boolean
  Compare To Constant4 : simulink/Logic and Bit Operations/Compare To Constant  relop=>=  const=-0.1  OutDataTypeStr=boolean
  Demux : Demux  Outputs=2
  safetyFlag : Outport
  wires:
  Demux/2 -> AND/2
  Demux/1 -> AND/1
  AND/1 -> safetyFlag/1
  errors/1 -> Compare To Constant4/1
  Compare To Constant4/1 -> Demux/1

== system gg_plus_lc_platoon/p2/Subsystem1/steadyState ==
  u : Inport
  AND : Logic  IconShape=distinctive  AllPortsSameDT=off  OutDataTypeStr=boolean
  Abs2 : Abs
  Compare To Constant2 : simulink/Logic and Bit Operations/Compare To Constant  relop=<=  const=0.2  OutDataTypeStr=boolean
  Demux : Demux  Outputs=2
  Mux : Mux  Inputs=2
  Transport Delay2 : TransportDelay
  ssFlag : Outport
  wires:
  u/1 -> Transport Delay2/1, Mux/2
  Abs2/1 -> Compare To Constant2/1
  Demux/1 -> AND/1
  Transport Delay2/1 -> Mux/1
  AND/1 -> ssFlag/1
  Compare To Constant2/1 -> Demux/1
  Mux/1 -> Abs2/1
  Demux/2 -> AND/2

== system gg_plus_lc_platoon/p2/Virtual Vehicle Following/Compute Errors ==
  xf : Inport
  vf : Inport  Port=2
  xl : Inport  Port=3
  vl : Inport  Port=4
  extraSpace : Inport  Port=5
  velFilterReset : Inport  Port=6
  Compare To Constant : simulink/Logic and Bit Operations/Compare To Constant  relop=<=  const=0  OutDataTypeStr=boolean
  Demux : Demux  Outputs=2
  Demux1 : Demux  Outputs=2
  Gain3 : Gain  Gain=velFilterGain/10
  Integrator : Integrator  InitialCondition=[h d0]
  Integrator1 : Integrator  ExternalReset=rising  InitialCondition=vx0
  Multiply : Product
  Mux : Mux  Inputs=2
  Mux1 : Mux  Inputs=2
  Product : Product
  Saturation : Saturate  UpperLimit=maxAcceleration  LowerLimit=minAcceleration
  Saturation1 : Saturate  UpperLimit=hFilterSaturation  LowerLimit=-hFilterSaturation
  Sum : Sum  Inputs=-+|
  Sum1 : Sum  Inputs=++|
  Sum2 : Sum  Inputs=+-|
  Sum3 : Sum  Inputs=|++
  Sum4 : Sum  Inputs=-+|
  Sum5 : Sum  Inputs=|+-
  Sum6 : Sum  Inputs=+-|
  Sum7 : Sum  Inputs=|++
  Sum8 : Sum  Inputs=|+-
  Switch : Switch  Criteria=u2 > Threshold
  d0 : Constant  Value=d0
  d0Lc : Constant  Value=d0Lc
  h : Constant  Value=h
  hFilterGain : Gain  Gain=hFilterGain
  hLc : Constant  Value=hLc
  vLen : Constant  Value=lr+lf
  eh : Outport
  ev : Outport  Port=2
  "gap " : Outport  Port=3
  unsafeFlag : Outport  Port=4
  wires:
  velFilterReset/1 -> Integrator1/2
  xl/1 -> Sum/2
  Sum6/1 -> Compare To Constant/1
  Mux/1 -> Demux1/1, Switch/3  "min safe gap"
  Sum7/1 -> Sum6/2  "safe  gap"
  Mux1/1 -> Switch/1
  d0/1 -> Mux/2
  Integrator/1 -> Demux/1, Sum5/2
  Demux1/1 -> Product/2
  Compare To Constant/1 -> unsafeFlag/1
  Sum2/1 -> eh/1
  extraSpace/1 -> Switch/2
  Product/1 -> Sum7/1
  h/1 -> Mux/1
  Sum3/1 -> Sum2/2  "desired  gap"
  Sum1/1 -> Sum/1  "x (front bumber)"
  vf/1 -> Sum4/1, Product/1, Multiply/1
  Sum5/1 -> hFilterGain/1
  Switch/1 -> Sum5/1
  Demux/2 -> Sum3/2
  vLen/1 -> Sum1/1
  hLc/1 -> Mux1/1
  Demux1/2 -> Sum7/2
  Multiply/1 -> Sum3/1
  Sum/1 -> Sum6/1, "gap "/1, Sum2/1  "gap"
  xf/1 -> Sum1/2
  Demux/1 -> Multiply/2
  hFilterGain/1 -> Saturation1/1
  d0Lc/1 -> Mux1/2
  Sum4/1 -> ev/1
  Integrator1/1 -> Sum4/2, Sum8/2
  Gain3/1 -> Saturation/1
  Sum8/1 -> Gain3/1
  Saturation/1 -> Integrator1/1
  vl/1 -> Sum8/1
  Saturation1/1 -> Integrator/1

== system gg_plus_lc_platoon/p2/Virtual Vehicle Following/Velocity Control Free Flow ==
  ev : Inport
  realInput : Inport  Port=2
  intReset : Inport  Port=3
  Anti-windup gain : Gain  Gain=velKp/velKi
  Integrator2 : Integrator  ExternalReset=falling
  Sum1 : Sum  Inputs=|-+
  Sum2 : Sum  Inputs=-+|
  Sum3 : Sum  Inputs=|++
  velKi : Gain  Gain=velKi
  velKp : Gain  Gain=velKp
  u : Outport
  wires:
  Sum2/1 -> Integrator2/1
  Sum1/1 -> Anti-windup gain/1
  realInput/1 -> Sum1/1
  Anti-windup gain/1 -> Sum2/1
  Sum3/1 -> u/1, Sum1/2
  intReset/1 -> Integrator2/2
  Integrator2/1 -> Sum3/1
  velKi/1 -> Sum2/2
  velKp/1 -> Sum3/2
  ev/1 -> velKp/1, velKi/1

== system gg_plus_lc_platoon/p2/Virtual Vehicle Following/Velocity Control Min ==
  note: Velocity control
  ev : Inport
  intReset : Inport  Port=2
  Integrator2 : Integrator  ExternalReset=rising
  Sum3 : Sum
  velKi : Gain  Gain=velKi
  velKp : Gain  Gain=velKp
  u : Outport
  wires:
  Integrator2/1 -> velKi/1
  velKi/1 -> Sum3/2
  Sum3/1 -> u/1
  velKp/1 -> Sum3/1
  ev/1 -> velKp/1, Integrator2/1
  intReset/1 -> Integrator2/2

== system gg_plus_lc_platoon/p2/Virtual Vehicle Following/Virtual Leader Following ==
  eh : Inport
  ev : Inport  Port=2
  realInput : Inport  Port=3
  intReset : Inport  Port=4
  Anti-windup gain : Gain  Gain=sqrt(Ki/Kd)
  Gain : Gain  Gain=10
  Integrator : Integrator  ExternalReset=rising
  Integrator2 : Integrator  ExternalReset=rising
  Kd : Gain  Gain=Kd
  Ki : Gain  Gain=Ki
  Kp : Gain  Gain=Kp
  Saturation1 : Saturate  UpperLimit=maxHeadwayError  LowerLimit=minHeadwayError
  Scope : Scope  NumInputPorts=4
  Scope1 : Scope  NumInputPorts=2
  Sum : Sum  Inputs=|-+
  Sum1 : Sum  Inputs=+++
  Sum5 : Sum  Inputs=-+|
  Sum9 : Sum  Inputs=|+-
  u : Outport
  wires:
  Saturation1/1 -> Sum9/1, Scope1/1
  Sum9/1 -> Gain/1
  Gain/1 -> Integrator2/1
  ev/1 -> Kd/1
  Ki/1 -> Sum5/2
  Anti-windup gain/1 -> Sum5/1
  Sum5/1 -> Integrator/1
  Integrator/1 -> Sum1/1, Scope/1
  Kp/1 -> Scope/2, Sum1/2
  Kd/1 -> Scope/3, Sum1/3
  Integrator2/1 -> Kp/1, Ki/1, Scope1/2, Sum9/2
  eh/1 -> Saturation1/1
  Sum1/1 -> Sum/2, u/1, Scope/4
  realInput/1 -> Sum/1
  Sum/1 -> Anti-windup gain/1
  intReset/1 -> Integrator/2, Integrator2/2

== system gg_plus_lc_platoon/p2/findLeader/Subsystem ==
  ego : Inport
  all : Inport  Port=2
  Enable : EnablePort
  MATLAB Function : MATLAB Function  TreatAsAtomicUnit=on
  idx : Outport  InitialOutput=1
  wires:
  ego/1 -> MATLAB Function/1(ego)
  MATLAB Function/1(leaderIdx) -> idx/1
  all/1 -> MATLAB Function/2(allVehicles)

== system gg_plus_lc_platoon/p2/findLeader/farAwayVeh ==
  ego : Inport  OutDataTypeStr=Bus: vehStatesBus
  Bus Creator : BusCreator  Inputs=6  OutDataTypeStr=Bus: vehStatesBus  NonVirtualBus=on
  Bus Selector : BusSelector  OutputSignals=X,Y,Xdot,psi,u,delta
  Constant : Constant  Value=1000
  Sum : Sum  Inputs=++|
  Out1 : Outport  OutDataTypeStr=Bus: vehStatesBus
  wires:
  Bus Creator/1 -> Out1/1
  Constant/1 -> Sum/1
  Bus Selector/1 -> Sum/2  "<X>"
  ego/1 -> Bus Selector/1
  Sum/1 -> Bus Creator/1  "X"
  Bus Selector/2 -> Bus Creator/2  "<Y>"
  Bus Selector/3 -> Bus Creator/3  "<Xdot>"
  Bus Selector/4 -> Bus Creator/4  "<psi>"
  Bus Selector/5 -> Bus Creator/5  "<u>"
  Bus Selector/6 -> Bus Creator/6  "<delta>"

== system gg_plus_lc_platoon/p2/followerErrors/gapToFollower ==
  xf : Inport
  vf : Inport  Port=2
  xl : Inport  Port=3
  Multiply : Product
  Sum : Sum  Inputs=-+|
  Sum1 : Sum  Inputs=++|
  Sum2 : Sum  Inputs=+-|
  Sum3 : Sum  Inputs=|++
  d0 : Constant  Value=d0
  h : Constant  Value=h
  vLen : Constant  Value=lr+lf
  eh : Outport
  "gap " : Outport  Port=2
  wires:
  vLen/1 -> Sum1/1
  Multiply/1 -> Sum3/1
  Sum/1 -> "gap "/1, Sum2/1  "gap"
  xf/1 -> Sum1/2
  Sum3/1 -> Sum2/2  "desired  gap"
  vf/1 -> Multiply/1
  Sum1/1 -> Sum/1  "x (front bumber)"
  xl/1 -> Sum/2
  Sum2/1 -> eh/1
  h/1 -> Multiply/2  "time headway"
  d0/1 -> Sum3/2  "gap at  standstill"

== system gg_plus_lc_platoon/p2/safeErrors/Triggered Subsystem1 ==
  Trigger : TriggerPort  VariantControl=Variant
  Constant : Constant  Value=true  OutDataTypeStr=boolean
  Out1 : Outport  OutDataTypeStr=boolean  InitialOutput=0
  wires:
  Constant/1 -> Out1/1

== system gg_plus_lc_platoon/p3/Lateral Control/Full State Observer ==
  note: yhat
  note: xhat
  measuredOutputs : Inport
  delta : Inport  Port=2
  Add1 : Sum  Inputs=|-+
  Gain : Gain  Gain=B  Multiplication=Matrix(K*u)
  Gain1 : Gain  Gain=C  Multiplication=Matrix(K*u)
  Gain2 : Gain  Gain=L  Multiplication=Matrix(K*u)
  Gain3 : Gain  Gain=A  Multiplication=Matrix(K*u)
  Integrator : Integrator  InitialCondition=[y0; 0; 0; 0]
  Signal Specification : SignalSpecification  Dimensions=[size(C,1) 1]
  Sum : Sum  Inputs=+++
  xhat : Outport
  wires:
  Gain2/1 -> Sum/1
  Signal Specification/1 -> Gain2/1
  Gain3/1 -> Sum/2
  Gain/1 -> Sum/3
  delta/1 -> Gain/1
  measuredOutputs/1 -> Add1/2
  Sum/1 -> Integrator/1
  Gain1/1 -> Add1/1
  Integrator/1 -> Gain1/1, Gain3/1, xhat/1
  Add1/1 -> Signal Specification/1

== system gg_plus_lc_platoon/p3/Lateral Control/Triggered Subsystem1 ==
  In1 : Inport
  Trigger : TriggerPort  VariantControl=Variant
  Out1 : Outport  InitialOutput=y0
  wires:
  In1/1 -> Out1/1

== system gg_plus_lc_platoon/p3/Regular Vehicle Following/Compute Errors ==
  xf : Inport
  vf : Inport  Port=2
  xl : Inport  Port=3
  vl : Inport  Port=4
  extraSpaceFlag : Inport  Port=5
  velFilterReset : Inport  Port=6
  Compare To Constant : simulink/Logic and Bit Operations/Compare To Constant  relop=<  const=-0.1  OutDataTypeStr=boolean
  Demux : Demux  Outputs=2
  Demux1 : Demux  Outputs=2
  Gain3 : Gain  Gain=velFilterGain
  Integrator : Integrator  InitialCondition=[h d0]
  Integrator1 : Integrator  ExternalReset=rising  InitialCondition=vx0
  Multiply : Product
  Mux : Mux  Inputs=2
  Mux1 : Mux  Inputs=2
  Product : Product
  Saturation : Saturate  UpperLimit=maxAcceleration  LowerLimit=minAcceleration
  Saturation1 : Saturate  UpperLimit=hFilterSaturation  LowerLimit=-hFilterSaturation
  Sum : Sum  Inputs=-+|
  Sum1 : Sum  Inputs=++|
  Sum2 : Sum  Inputs=+-|
  Sum3 : Sum  Inputs=|++
  Sum4 : Sum  Inputs=-+|
  Sum5 : Sum  Inputs=|+-
  Sum6 : Sum  Inputs=+-|
  Sum7 : Sum  Inputs=|++
  Sum8 : Sum  Inputs=|+-
  Switch : Switch  Criteria=u2 > Threshold
  d0 : Constant  Value=d0
  d0Lc : Constant  Value=d0Lc
  h : Constant  Value=h
  hFilterGain : Gain  Gain=hFilterGain
  hLc : Constant  Value=hLc
  vLen : Constant  Value=lr+lf
  eh : Outport
  ev : Outport  Port=2
  "gap " : Outport  Port=3
  unsafeFlag : Outport  Port=4
  wires:
  Sum8/1 -> Gain3/1
  Integrator1/1 -> Sum4/2, Sum8/2
  Saturation/1 -> Integrator1/1
  Gain3/1 -> Saturation/1
  Sum4/1 -> ev/1
  vl/1 -> Sum8/1
  d0Lc/1 -> Mux1/2
  hFilterGain/1 -> Saturation1/1
  Demux/1 -> Multiply/2
  xf/1 -> Sum1/2
  Sum/1 -> Sum2/1, "gap "/1, Sum6/1  "gap"
  Multiply/1 -> Sum3/1
  Demux1/2 -> Sum7/2
  hLc/1 -> Mux1/1
  vLen/1 -> Sum1/1
  Demux/2 -> Sum3/2
  Switch/1 -> Sum5/1
  Sum5/1 -> hFilterGain/1
  vf/1 -> Multiply/1, Product/1, Sum4/1
  Sum1/1 -> Sum/1  "x (front bumber)"
  Sum3/1 -> Sum2/2  "desired  gap"
  h/1 -> Mux/1
  Product/1 -> Sum7/1
  xl/1 -> Sum/2
  extraSpaceFlag/1 -> Switch/2
  Sum2/1 -> eh/1
  Compare To Constant/1 -> unsafeFlag/1
  Demux1/1 -> Product/2
  Integrator/1 -> Sum5/2, Demux/1
  d0/1 -> Mux/2
  Mux1/1 -> Switch/1
  Sum7/1 -> Sum6/2  "safe  gap"
  Mux/1 -> Demux1/1, Switch/3  "min safe gap"
  Sum6/1 -> Compare To Constant/1
  velFilterReset/1 -> Integrator1/2
  Saturation1/1 -> Integrator/1

== system gg_plus_lc_platoon/p3/Regular Vehicle Following/Veh Following ==
  eh : Inport
  ev : Inport  Port=2
  realInput : Inport  Port=3
  intReset : Inport  Port=4
  Anti-windup gain : Gain  Gain=sqrt(Ki/Kd)
  Integrator : Integrator  ExternalReset=rising
  Kd : Gain  Gain=Kd
  Ki : Gain  Gain=Ki
  Kp : Gain  Gain=Kp
  Saturation1 : Saturate  UpperLimit=maxHeadwayError  LowerLimit=minHeadwayError
  Scope : Scope  NumInputPorts=4
  Sum : Sum  Inputs=|-+
  Sum1 : Sum  Inputs=+++
  Sum5 : Sum  Inputs=-+|
  u : Outport
  wires:
  intReset/1 -> Integrator/2
  ev/1 -> Kd/1
  Ki/1 -> Sum5/2
  Anti-windup gain/1 -> Sum5/1
  Sum5/1 -> Integrator/1
  Kp/1 -> Sum1/2, Scope/2
  Kd/1 -> Sum1/3, Scope/3
  Saturation1/1 -> Ki/1, Kp/1
  eh/1 -> Saturation1/1
  Sum1/1 -> u/1, Sum/2, Scope/4
  realInput/1 -> Sum/1
  Sum/1 -> Anti-windup gain/1
  Integrator/1 -> Scope/1, Sum1/1

== system gg_plus_lc_platoon/p3/Regular Vehicle Following/Velocity Control ==
  velocity : Inport
  realInput : Inport  Port=2
  intReset : Inport  Port=3
  Anti-windup gain : Gain  Gain=velKp/velKi
  Integrator2 : Integrator  ExternalReset=falling
  Sum : Sum  Inputs=|+-
  Sum1 : Sum  Inputs=|-+
  Sum2 : Sum  Inputs=-+|
  Sum3 : Sum  Inputs=|++
  freeFlowVel : Constant  Value=freeFlowVel
  velKi : Gain  Gain=velKi
  velKp : Gain  Gain=velKp
  u : Outport
  wires:
  Anti-windup gain/1 -> Sum2/1
  Sum/1 -> velKi/1, velKp/1
  velKp/1 -> Sum3/2
  velKi/1 -> Sum2/2
  Integrator2/1 -> Sum3/1
  velocity/1 -> Sum/2
  freeFlowVel/1 -> Sum/1
  intReset/1 -> Integrator2/2
  Sum3/1 -> Sum1/2, u/1
  realInput/1 -> Sum1/1
  Sum1/1 -> Anti-windup gain/1
  Sum2/1 -> Integrator2/1

== system gg_plus_lc_platoon/p3/Subsystem1/Triggered Subsystem1 ==
  Trigger : TriggerPort  VariantControl=Variant
  Constant : Constant  Value=true  OutDataTypeStr=boolean
  Out1 : Outport  OutDataTypeStr=boolean  InitialOutput=0
  wires:
  Constant/1 -> Out1/1

== system gg_plus_lc_platoon/p3/Subsystem1/safeErrors1 ==
  errors : Inport
  AND : Logic  IconShape=distinctive  AllPortsSameDT=off  OutDataTypeStr=boolean
  Compare To Constant4 : simulink/Logic and Bit Operations/Compare To Constant  relop=>=  const=-0.1  OutDataTypeStr=boolean
  Demux : Demux  Outputs=2
  safetyFlag : Outport
  wires:
  Compare To Constant4/1 -> Demux/1
  errors/1 -> Compare To Constant4/1
  AND/1 -> safetyFlag/1
  Demux/1 -> AND/1
  Demux/2 -> AND/2

== system gg_plus_lc_platoon/p3/Subsystem1/safeErrors2 ==
  errors : Inport
  AND : Logic  IconShape=distinctive  AllPortsSameDT=off  OutDataTypeStr=boolean
  Compare To Constant4 : simulink/Logic and Bit Operations/Compare To Constant  relop=>=  const=-0.1  OutDataTypeStr=boolean
  Demux : Demux  Outputs=2
  safetyFlag : Outport
  wires:
  Demux/2 -> AND/2
  Demux/1 -> AND/1
  AND/1 -> safetyFlag/1
  errors/1 -> Compare To Constant4/1
  Compare To Constant4/1 -> Demux/1

== system gg_plus_lc_platoon/p3/Subsystem1/steadyState ==
  u : Inport
  AND : Logic  IconShape=distinctive  AllPortsSameDT=off  OutDataTypeStr=boolean
  Abs2 : Abs
  Compare To Constant2 : simulink/Logic and Bit Operations/Compare To Constant  relop=<=  const=0.2  OutDataTypeStr=boolean
  Demux : Demux  Outputs=2
  Mux : Mux  Inputs=2
  Transport Delay2 : TransportDelay
  ssFlag : Outport
  wires:
  u/1 -> Transport Delay2/1, Mux/2
  Abs2/1 -> Compare To Constant2/1
  Demux/1 -> AND/1
  Transport Delay2/1 -> Mux/1
  AND/1 -> ssFlag/1
  Compare To Constant2/1 -> Demux/1
  Mux/1 -> Abs2/1
  Demux/2 -> AND/2

== system gg_plus_lc_platoon/p3/Virtual Vehicle Following/Compute Errors ==
  xf : Inport
  vf : Inport  Port=2
  xl : Inport  Port=3
  vl : Inport  Port=4
  extraSpace : Inport  Port=5
  velFilterReset : Inport  Port=6
  Compare To Constant : simulink/Logic and Bit Operations/Compare To Constant  relop=<=  const=0  OutDataTypeStr=boolean
  Demux : Demux  Outputs=2
  Demux1 : Demux  Outputs=2
  Gain3 : Gain  Gain=velFilterGain/10
  Integrator : Integrator  InitialCondition=[h d0]
  Integrator1 : Integrator  ExternalReset=rising  InitialCondition=vx0
  Multiply : Product
  Mux : Mux  Inputs=2
  Mux1 : Mux  Inputs=2
  Product : Product
  Saturation : Saturate  UpperLimit=maxAcceleration  LowerLimit=minAcceleration
  Saturation1 : Saturate  UpperLimit=hFilterSaturation  LowerLimit=-hFilterSaturation
  Sum : Sum  Inputs=-+|
  Sum1 : Sum  Inputs=++|
  Sum2 : Sum  Inputs=+-|
  Sum3 : Sum  Inputs=|++
  Sum4 : Sum  Inputs=-+|
  Sum5 : Sum  Inputs=|+-
  Sum6 : Sum  Inputs=+-|
  Sum7 : Sum  Inputs=|++
  Sum8 : Sum  Inputs=|+-
  Switch : Switch  Criteria=u2 > Threshold
  d0 : Constant  Value=d0
  d0Lc : Constant  Value=d0Lc
  h : Constant  Value=h
  hFilterGain : Gain  Gain=hFilterGain
  hLc : Constant  Value=hLc
  vLen : Constant  Value=lr+lf
  eh : Outport
  ev : Outport  Port=2
  "gap " : Outport  Port=3
  unsafeFlag : Outport  Port=4
  wires:
  velFilterReset/1 -> Integrator1/2
  xl/1 -> Sum/2
  Sum6/1 -> Compare To Constant/1
  Mux/1 -> Demux1/1, Switch/3  "min safe gap"
  Sum7/1 -> Sum6/2  "safe  gap"
  Mux1/1 -> Switch/1
  d0/1 -> Mux/2
  Integrator/1 -> Demux/1, Sum5/2
  Demux1/1 -> Product/2
  Compare To Constant/1 -> unsafeFlag/1
  Sum2/1 -> eh/1
  extraSpace/1 -> Switch/2
  Product/1 -> Sum7/1
  h/1 -> Mux/1
  Sum3/1 -> Sum2/2  "desired  gap"
  Sum1/1 -> Sum/1  "x (front bumber)"
  vf/1 -> Sum4/1, Product/1, Multiply/1
  Sum5/1 -> hFilterGain/1
  Switch/1 -> Sum5/1
  Demux/2 -> Sum3/2
  vLen/1 -> Sum1/1
  hLc/1 -> Mux1/1
  Demux1/2 -> Sum7/2
  Multiply/1 -> Sum3/1
  Sum/1 -> Sum6/1, "gap "/1, Sum2/1  "gap"
  xf/1 -> Sum1/2
  Demux/1 -> Multiply/2
  hFilterGain/1 -> Saturation1/1
  d0Lc/1 -> Mux1/2
  Sum4/1 -> ev/1
  Integrator1/1 -> Sum4/2, Sum8/2
  Gain3/1 -> Saturation/1
  Sum8/1 -> Gain3/1
  Saturation/1 -> Integrator1/1
  vl/1 -> Sum8/1
  Saturation1/1 -> Integrator/1

== system gg_plus_lc_platoon/p3/Virtual Vehicle Following/Velocity Control Free Flow ==
  ev : Inport
  realInput : Inport  Port=2
  intReset : Inport  Port=3
  Anti-windup gain : Gain  Gain=velKp/velKi
  Integrator2 : Integrator  ExternalReset=falling
  Sum1 : Sum  Inputs=|-+
  Sum2 : Sum  Inputs=-+|
  Sum3 : Sum  Inputs=|++
  velKi : Gain  Gain=velKi
  velKp : Gain  Gain=velKp
  u : Outport
  wires:
  Sum2/1 -> Integrator2/1
  Sum1/1 -> Anti-windup gain/1
  realInput/1 -> Sum1/1
  Anti-windup gain/1 -> Sum2/1
  Sum3/1 -> u/1, Sum1/2
  intReset/1 -> Integrator2/2
  Integrator2/1 -> Sum3/1
  velKi/1 -> Sum2/2
  velKp/1 -> Sum3/2
  ev/1 -> velKp/1, velKi/1

== system gg_plus_lc_platoon/p3/Virtual Vehicle Following/Velocity Control Min ==
  note: Velocity control
  ev : Inport
  intReset : Inport  Port=2
  Integrator2 : Integrator  ExternalReset=rising
  Sum3 : Sum
  velKi : Gain  Gain=velKi
  velKp : Gain  Gain=velKp
  u : Outport
  wires:
  Integrator2/1 -> velKi/1
  velKi/1 -> Sum3/2
  Sum3/1 -> u/1
  velKp/1 -> Sum3/1
  ev/1 -> velKp/1, Integrator2/1
  intReset/1 -> Integrator2/2
